simulink model "static_wind_field"  (R2020b)
settings: Solver=VariableStepAuto  StartTime=0.0  StopTime=10.0  RelTol=1e-3
settings Model: Creator=Dogukan  LastModifiedBy=Dogukan

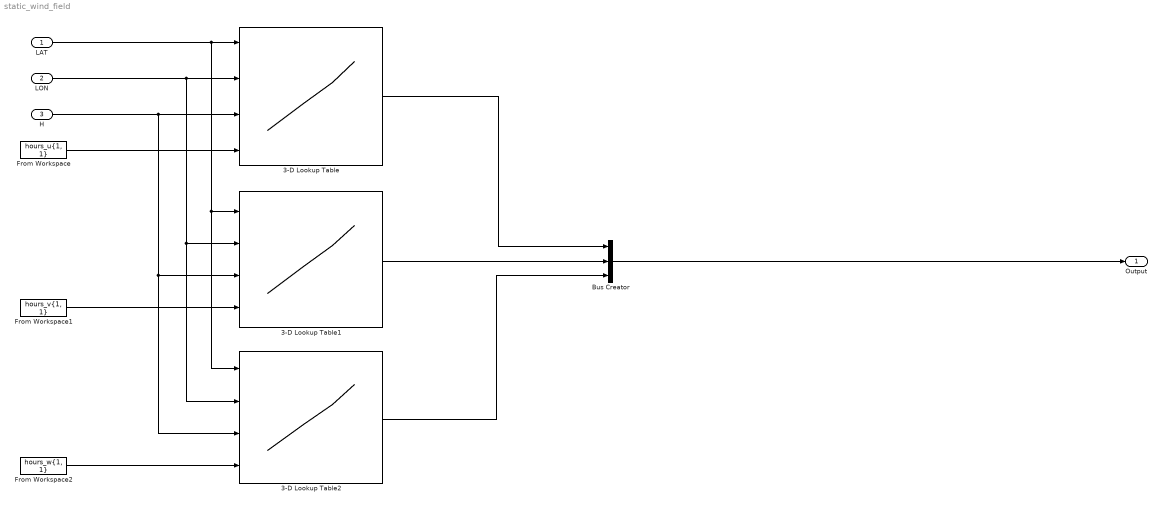
== system static_wind_field ==
  LAT : Inport
  LON : Inport  Port=2
  H : Inport  Port=3
  3-D Lookup Table : Lookup_n-D  NumberOfTableDimensions=3  BreakpointsForDimension3=[5, 7]  TableSource=Input port  Table=reshape(repmat([4 5 6;16 19 20;10 18 23],1,2),[3,3,2])  ExtrapMethod=Clip  InternalRulePriority=Speed  RndMeth=Simplest  InputSameDT=on
      settings: InputPortMap=u0,u1,u2,p221
  3-D Lookup Table1 : Lookup_n-D  NumberOfTableDimensions=3  BreakpointsForDimension3=[5, 7]  TableSource=Input port  Table=reshape(repmat([4 5 6;16 19 20;10 18 23],1,2),[3,3,2])  ExtrapMethod=Clip  InternalRulePriority=Speed  RndMeth=Simplest  InputSameDT=on
      settings: InputPortMap=u0,u1,u2,p221
  3-D Lookup Table2 : Lookup_n-D  NumberOfTableDimensions=3  BreakpointsForDimension3=[5, 7]  TableSource=Input port  Table=reshape(repmat([4 5 6;16 19 20;10 18 23],1,2),[3,3,2])  ExtrapMethod=Clip  InternalRulePriority=Speed  RndMeth=Simplest  InputSameDT=on
      settings: InputPortMap=u0,u1,u2,p221
  Bus Creator : BusCreator  Inputs=3
  From Workspace : FromWorkspace  VariableName=hours_u{1, 1}
  From Workspace1 : FromWorkspace  VariableName=hours_v{1, 1}
  From Workspace2 : FromWorkspace  VariableName=hours_w{1, 1}
  Output : Outport
  wires:
  LAT/1 -> 3-D Lookup Table2/1, 3-D Lookup Table1/1, 3-D Lookup Table/1
  LON/1 -> 3-D Lookup Table2/2, 3-D Lookup Table1/2, 3-D Lookup Table/2
  H/1 -> 3-D Lookup Table2/3, 3-D Lookup Table1/3, 3-D Lookup Table/3
  3-D Lookup Table/1 -> Bus Creator/1
  3-D Lookup Table1/1 -> Bus Creator/2
  Bus Creator/1 -> Output/1
  3-D Lookup Table2/1 -> Bus Creator/3
  From Workspace/1 -> 3-D Lookup Table/4
  From Workspace1/1 -> 3-D Lookup Table1/4
  From Workspace2/1 -> 3-D Lookup Table2/4
